simulink model "TST_Rail_MonMeUn"  (R2016b)
settings: Solver=FixedStepDiscrete  StartTime=0.0  StopTime=simTime  FixedStep=sampleTime  RelTol=1e-3
values from neighbouring files (symbols this model uses):
  testCase = 1    [initTST_Rail_MonMeUn_001.m]    (also in initTST_Rail_MonMeUn_002.m = 2; initTST_Rail_MonMeUn_003.m = 3; initTST_Rail_MonMeUn_004.m = 4; initTST_Rail_MonMeUn_005.m = 5)
libraries: simulink x91, UnitTest_Lib x81
(part 5 of 5)

== system TST_Rail_MonMeUn/compareSignals/Requirement_003/specifyOutputs ==
  sig_Req_Bus : Inport
  sig_Result_Bus : Inport  Port=2
  AndN : Logic  Inputs=9
  BS_Req : BusSelector  OutputSignals=testSig_DFC_RailMeUn0_DSM,testSig_DFC_RailMeUn2_DSM,testSig_DFC_RailMeUn22_DSM,testSig_DFC_RailMeUn3_DSM,testSig_DFC_RailMeUn4_DSM,testSig_DFC_RailMeUn42_DSM,testSig_DFC_RailMeUn7_DSM,testSig_DFC_RailMeUn8_DSM,testSig_DFC_RailMeUn10_DSM
  BS_Result : BusSelector  OutputSignals=DFC_RailMeUn0_DSM,DFC_RailMeUn2_DSM,DFC_RailMeUn22_DSM,DFC_RailMeUn3_DSM,DFC_RailMeUn4_DSM,DFC_RailMeUn42_DSM,DFC_RailMeUn7_DSM,DFC_RailMeUn8_DSM,DFC_RailMeUn10_DSM
  Bitwise_And{1..9} (9 alike) : simulink/Logic and Bit Operations/Bitwise Operator  logicop=AND  UseBitMask=off  BitMask=bin2dec('11011001')  BitMaskRealWorld=Stored Integer
  Scope : Scope  NumInputPorts=9
  Scope{1..9} (9 alike) : Scope  NumInputPorts=2
  cmp_{1..9} (9 alike) : UnitTest_Lib/RoughlyEqual  slope=0.1
  result_tws : ToWorkspace  VariableName=spec_result_003
  tws_1 : ToWorkspace  VariableName=spec_req_003_001
  tws_2 : ToWorkspace  VariableName=spec_req_003_002
  tws_3 : ToWorkspace  VariableName=spec_req_003_003
  tws_4 : ToWorkspace  VariableName=spec_req_003_004
  tws_5 : ToWorkspace  VariableName=spec_req_003_005
  tws_6 : ToWorkspace  VariableName=spec_req_003_006
  tws_7 : ToWorkspace  VariableName=spec_req_003_007
  tws_8 : ToWorkspace  VariableName=spec_req_003_008
  tws_9 : ToWorkspace  VariableName=spec_req_003_009
  result : Outport
  wires:
  sig_Req_Bus/1 -> BS_Req/1
  sig_Result_Bus/1 -> BS_Result/1
  AndN/1 -> result/1, result_tws/1
  BS_Req/1 -> cmp_1/1, Scope1/1  "<testSig_DFC_RailMeUn0_DSM>"
  BS_Result/1 -> cmp_1/2, Scope1/2  "<DFC_RailMeUn0_DSM>"
  cmp_1/1 -> Bitwise_And1/1
  Bitwise_And1/1 -> tws_1/1, AndN/1, Scope/1
  BS_Req/2 -> cmp_2/1, Scope2/1  "<testSig_DFC_RailMeUn2_DSM>"
  BS_Result/2 -> cmp_2/2, Scope2/2  "<DFC_RailMeUn2_DSM>"
  cmp_2/1 -> Bitwise_And2/1
  Bitwise_And2/1 -> tws_2/1, AndN/2, Scope/2
  BS_Req/3 -> cmp_3/1, Scope3/1  "<testSig_DFC_RailMeUn22_DSM>"
  BS_Result/3 -> cmp_3/2, Scope3/2  "<DFC_RailMeUn22_DSM>"
  cmp_3/1 -> Bitwise_And3/1
  Bitwise_And3/1 -> tws_3/1, AndN/3, Scope/3
  BS_Req/4 -> cmp_4/1, Scope4/1  "<testSig_DFC_RailMeUn3_DSM>"
  BS_Result/4 -> cmp_4/2, Scope4/2  "<DFC_RailMeUn3_DSM>"
  cmp_4/1 -> Bitwise_And4/1
  Bitwise_And4/1 -> tws_4/1, AndN/4, Scope/4
  BS_Req/5 -> cmp_5/1, Scope5/1  "<testSig_DFC_RailMeUn4_DSM>"
  BS_Result/5 -> cmp_5/2, Scope5/2  "<DFC_RailMeUn4_DSM>"
  cmp_5/1 -> Bitwise_And5/1
  Bitwise_And5/1 -> tws_5/1, AndN/5, Scope/5
  BS_Req/6 -> cmp_6/1, Scope6/1  "<testSig_DFC_RailMeUn42_DSM>"
  BS_Result/6 -> cmp_6/2, Scope6/2  "<DFC_RailMeUn42_DSM>"
  cmp_6/1 -> Bitwise_And6/1
  Bitwise_And6/1 -> tws_6/1, AndN/6, Scope/6
  BS_Req/7 -> cmp_7/1, Scope7/1  "<testSig_DFC_RailMeUn7_DSM>"
  BS_Result/7 -> cmp_7/2, Scope7/2  "<DFC_RailMeUn7_DSM>"
  cmp_7/1 -> Bitwise_And7/1
  Bitwise_And7/1 -> tws_7/1, AndN/7, Scope/7
  BS_Req/8 -> cmp_8/1, Scope8/1  "<testSig_DFC_RailMeUn8_DSM>"
  BS_Result/8 -> cmp_8/2, Scope8/2  "<DFC_RailMeUn8_DSM>"
  cmp_8/1 -> Bitwise_And8/1
  Bitwise_And8/1 -> tws_8/1, AndN/8, Scope/8
  BS_Req/9 -> cmp_9/1, Scope9/1  "<testSig_DFC_RailMeUn10_DSM>"
  BS_Result/9 -> cmp_9/2, Scope9/2  "<DFC_RailMeUn10_DSM>"
  cmp_9/1 -> Bitwise_And9/1
  Bitwise_And9/1 -> tws_9/1, AndN/9, Scope/9

== system TST_Rail_MonMeUn/compareSignals/Requirement_004/specifyOutputs ==
  sig_Req_Bus : Inport
  sig_Result_Bus : Inport  Port=2
  AndN : Logic  Inputs=9
  BS_Req : BusSelector  OutputSignals=testSig_DFC_RailMeUn0_DSM,testSig_DFC_RailMeUn2_DSM,testSig_DFC_RailMeUn22_DSM,testSig_DFC_RailMeUn3_DSM,testSig_DFC_RailMeUn4_DSM,testSig_DFC_RailMeUn42_DSM,testSig_DFC_RailMeUn7_DSM,testSig_DFC_RailMeUn8_DSM,testSig_DFC_RailMeUn10_DSM
  BS_Result : BusSelector  OutputSignals=DFC_RailMeUn0_DSM,DFC_RailMeUn2_DSM,DFC_RailMeUn22_DSM,DFC_RailMeUn3_DSM,DFC_RailMeUn4_DSM,DFC_RailMeUn42_DSM,DFC_RailMeUn7_DSM,DFC_RailMeUn8_DSM,DFC_RailMeUn10_DSM
  Bitwise_And{1..9} (9 alike) : simulink/Logic and Bit Operations/Bitwise Operator  logicop=AND  UseBitMask=off  BitMask=bin2dec('11011001')  BitMaskRealWorld=Stored Integer
  Scope : Scope  NumInputPorts=9
  Scope{1..9} (9 alike) : Scope  NumInputPorts=2
  cmp_{1..9} (9 alike) : UnitTest_Lib/RoughlyEqual  slope=0.1
  result_tws : ToWorkspace  VariableName=spec_result_004
  tws_1 : ToWorkspace  VariableName=spec_req_004_001
  tws_2 : ToWorkspace  VariableName=spec_req_004_002
  tws_3 : ToWorkspace  VariableName=spec_req_004_003
  tws_4 : ToWorkspace  VariableName=spec_req_004_004
  tws_5 : ToWorkspace  VariableName=spec_req_004_005
  tws_6 : ToWorkspace  VariableName=spec_req_004_006
  tws_7 : ToWorkspace  VariableName=spec_req_004_007
  tws_8 : ToWorkspace  VariableName=spec_req_004_008
  tws_9 : ToWorkspace  VariableName=spec_req_004_009
  result : Outport
  wires:
  sig_Req_Bus/1 -> BS_Req/1
  sig_Result_Bus/1 -> BS_Result/1
  AndN/1 -> result/1, result_tws/1
  BS_Req/1 -> cmp_1/1, Scope1/1  "<testSig_DFC_RailMeUn0_DSM>"
  BS_Result/1 -> cmp_1/2, Scope1/2  "<DFC_RailMeUn0_DSM>"
  cmp_1/1 -> Bitwise_And1/1
  Bitwise_And1/1 -> tws_1/1, AndN/1, Scope/1
  BS_Req/2 -> cmp_2/1, Scope2/1  "<testSig_DFC_RailMeUn2_DSM>"
  BS_Result/2 -> cmp_2/2, Scope2/2  "<DFC_RailMeUn2_DSM>"
  cmp_2/1 -> Bitwise_And2/1
  Bitwise_And2/1 -> tws_2/1, AndN/2, Scope/2
  BS_Req/3 -> cmp_3/1, Scope3/1  "<testSig_DFC_RailMeUn22_DSM>"
  BS_Result/3 -> cmp_3/2, Scope3/2  "<DFC_RailMeUn22_DSM>"
  cmp_3/1 -> Bitwise_And3/1
  Bitwise_And3/1 -> tws_3/1, AndN/3, Scope/3
  BS_Req/4 -> cmp_4/1, Scope4/1  "<testSig_DFC_RailMeUn3_DSM>"
  BS_Result/4 -> cmp_4/2, Scope4/2  "<DFC_RailMeUn3_DSM>"
  cmp_4/1 -> Bitwise_And4/1
  Bitwise_And4/1 -> tws_4/1, AndN/4, Scope/4
  BS_Req/5 -> cmp_5/1, Scope5/1  "<testSig_DFC_RailMeUn4_DSM>"
  BS_Result/5 -> cmp_5/2, Scope5/2  "<DFC_RailMeUn4_DSM>"
  cmp_5/1 -> Bitwise_And5/1
  Bitwise_And5/1 -> tws_5/1, AndN/5, Scope/5
  BS_Req/6 -> cmp_6/1, Scope6/1  "<testSig_DFC_RailMeUn42_DSM>"
  BS_Result/6 -> cmp_6/2, Scope6/2  "<DFC_RailMeUn42_DSM>"
  cmp_6/1 -> Bitwise_And6/1
  Bitwise_And6/1 -> tws_6/1, AndN/6, Scope/6
  BS_Req/7 -> cmp_7/1, Scope7/1  "<testSig_DFC_RailMeUn7_DSM>"
  BS_Result/7 -> cmp_7/2, Scope7/2  "<DFC_RailMeUn7_DSM>"
  cmp_7/1 -> Bitwise_And7/1
  Bitwise_And7/1 -> tws_7/1, AndN/7, Scope/7
  BS_Req/8 -> cmp_8/1, Scope8/1  "<testSig_DFC_RailMeUn8_DSM>"
  BS_Result/8 -> cmp_8/2, Scope8/2  "<DFC_RailMeUn8_DSM>"
  cmp_8/1 -> Bitwise_And8/1
  Bitwise_And8/1 -> tws_8/1, AndN/8, Scope/8
  BS_Req/9 -> cmp_9/1, Scope9/1  "<testSig_DFC_RailMeUn10_DSM>"
  BS_Result/9 -> cmp_9/2, Scope9/2  "<DFC_RailMeUn10_DSM>"
  cmp_9/1 -> Bitwise_And9/1
  Bitwise_And9/1 -> tws_9/1, AndN/9, Scope/9

== system TST_Rail_MonMeUn/compareSignals/Requirement_005/specifyOutputs ==
  sig_Req_Bus : Inport
  sig_Result_Bus : Inport  Port=2
  AndN : Logic  Inputs=9
  BS_Req : BusSelector  OutputSignals=testSig_DFC_RailMeUn0_DSM,testSig_DFC_RailMeUn2_DSM,testSig_DFC_RailMeUn22_DSM,testSig_DFC_RailMeUn3_DSM,testSig_DFC_RailMeUn4_DSM,testSig_DFC_RailMeUn42_DSM,testSig_DFC_RailMeUn7_DSM,testSig_DFC_RailMeUn8_DSM,testSig_DFC_RailMeUn10_DSM
  BS_Result : BusSelector  OutputSignals=DFC_RailMeUn0_DSM,DFC_RailMeUn2_DSM,DFC_RailMeUn22_DSM,DFC_RailMeUn3_DSM,DFC_RailMeUn4_DSM,DFC_RailMeUn42_DSM,DFC_RailMeUn7_DSM,DFC_RailMeUn8_DSM,DFC_RailMeUn10_DSM
  Bitwise_And{1..9} (9 alike) : simulink/Logic and Bit Operations/Bitwise Operator  logicop=AND  UseBitMask=off  BitMask=bin2dec('11011001')  BitMaskRealWorld=Stored Integer
  Scope : Scope  NumInputPorts=9
  Scope{1..9} (9 alike) : Scope  NumInputPorts=2
  cmp_{1..9} (9 alike) : UnitTest_Lib/RoughlyEqual  slope=0.1
  result_tws : ToWorkspace  VariableName=spec_result_005
  tws_1 : ToWorkspace  VariableName=spec_req_005_001
  tws_2 : ToWorkspace  VariableName=spec_req_005_002
  tws_3 : ToWorkspace  VariableName=spec_req_005_003
  tws_4 : ToWorkspace  VariableName=spec_req_005_004
  tws_5 : ToWorkspace  VariableName=spec_req_005_005
  tws_6 : ToWorkspace  VariableName=spec_req_005_006
  tws_7 : ToWorkspace  VariableName=spec_req_005_007
  tws_8 : ToWorkspace  VariableName=spec_req_005_008
  tws_9 : ToWorkspace  VariableName=spec_req_005_009
  result : Outport
  wires:
  sig_Req_Bus/1 -> BS_Req/1
  sig_Result_Bus/1 -> BS_Result/1
  AndN/1 -> result/1, result_tws/1
  BS_Req/1 -> cmp_1/1, Scope1/1  "<testSig_DFC_RailMeUn0_DSM>"
  BS_Result/1 -> cmp_1/2, Scope1/2  "<DFC_RailMeUn0_DSM>"
  cmp_1/1 -> Bitwise_And1/1
  Bitwise_And1/1 -> tws_1/1, AndN/1, Scope/1
  BS_Req/2 -> cmp_2/1, Scope2/1  "<testSig_DFC_RailMeUn2_DSM>"
  BS_Result/2 -> cmp_2/2, Scope2/2  "<DFC_RailMeUn2_DSM>"
  cmp_2/1 -> Bitwise_And2/1
  Bitwise_And2/1 -> tws_2/1, AndN/2, Scope/2
  BS_Req/3 -> cmp_3/1, Scope3/1  "<testSig_DFC_RailMeUn22_DSM>"
  BS_Result/3 -> cmp_3/2, Scope3/2  "<DFC_RailMeUn22_DSM>"
  cmp_3/1 -> Bitwise_And3/1
  Bitwise_And3/1 -> tws_3/1, AndN/3, Scope/3
  BS_Req/4 -> cmp_4/1, Scope4/1  "<testSig_DFC_RailMeUn3_DSM>"
  BS_Result/4 -> cmp_4/2, Scope4/2  "<DFC_RailMeUn3_DSM>"
  cmp_4/1 -> Bitwise_And4/1
  Bitwise_And4/1 -> tws_4/1, AndN/4, Scope/4
  BS_Req/5 -> cmp_5/1, Scope5/1  "<testSig_DFC_RailMeUn4_DSM>"
  BS_Result/5 -> cmp_5/2, Scope5/2  "<DFC_RailMeUn4_DSM>"
  cmp_5/1 -> Bitwise_And5/1
  Bitwise_And5/1 -> tws_5/1, AndN/5, Scope/5
  BS_Req/6 -> cmp_6/1, Scope6/1  "<testSig_DFC_RailMeUn42_DSM>"
  BS_Result/6 -> cmp_6/2, Scope6/2  "<DFC_RailMeUn42_DSM>"
  cmp_6/1 -> Bitwise_And6/1
  Bitwise_And6/1 -> tws_6/1, AndN/6, Scope/6
  BS_Req/7 -> cmp_7/1, Scope7/1  "<testSig_DFC_RailMeUn7_DSM>"
  BS_Result/7 -> cmp_7/2, Scope7/2  "<DFC_RailMeUn7_DSM>"
  cmp_7/1 -> Bitwise_And7/1
  Bitwise_And7/1 -> tws_7/1, AndN/7, Scope/7
  BS_Req/8 -> cmp_8/1, Scope8/1  "<testSig_DFC_RailMeUn8_DSM>"
  BS_Result/8 -> cmp_8/2, Scope8/2  "<DFC_RailMeUn8_DSM>"
  cmp_8/1 -> Bitwise_And8/1
  Bitwise_And8/1 -> tws_8/1, AndN/8, Scope/8
  BS_Req/9 -> cmp_9/1, Scope9/1  "<testSig_DFC_RailMeUn10_DSM>"
  BS_Result/9 -> cmp_9/2, Scope9/2  "<DFC_RailMeUn10_DSM>"
  cmp_9/1 -> Bitwise_And9/1
  Bitwise_And9/1 -> tws_9/1, AndN/9, Scope/9

== system TST_Rail_MonMeUn/compareSignals/Requirement_006/specifyOutputs ==
  sig_Req_Bus : Inport
  sig_Result_Bus : Inport  Port=2
  AndN : Logic  Inputs=9
  BS_Req : BusSelector  OutputSignals=testSig_DFC_RailMeUn0_DSM,testSig_DFC_RailMeUn2_DSM,testSig_DFC_RailMeUn22_DSM,testSig_DFC_RailMeUn3_DSM,testSig_DFC_RailMeUn4_DSM,testSig_DFC_RailMeUn42_DSM,testSig_DFC_RailMeUn7_DSM,testSig_DFC_RailMeUn8_DSM,testSig_DFC_RailMeUn10_DSM
  BS_Result : BusSelector  OutputSignals=DFC_RailMeUn0_DSM,DFC_RailMeUn2_DSM,DFC_RailMeUn22_DSM,DFC_RailMeUn3_DSM,DFC_RailMeUn4_DSM,DFC_RailMeUn42_DSM,DFC_RailMeUn7_DSM,DFC_RailMeUn8_DSM,DFC_RailMeUn10_DSM
  Bitwise_And{1..9} (9 alike) : simulink/Logic and Bit Operations/Bitwise Operator  logicop=AND  UseBitMask=off  BitMask=bin2dec('11011001')  BitMaskRealWorld=Stored Integer
  Scope : Scope  NumInputPorts=9
  Scope{1..9} (9 alike) : Scope  NumInputPorts=2
  cmp_{1..9} (9 alike) : UnitTest_Lib/RoughlyEqual  slope=0.1
  result_tws : ToWorkspace  VariableName=spec_result_006
  tws_1 : ToWorkspace  VariableName=spec_req_006_001
  tws_2 : ToWorkspace  VariableName=spec_req_006_002
  tws_3 : ToWorkspace  VariableName=spec_req_006_003
  tws_4 : ToWorkspace  VariableName=spec_req_006_004
  tws_5 : ToWorkspace  VariableName=spec_req_006_005
  tws_6 : ToWorkspace  VariableName=spec_req_006_006
  tws_7 : ToWorkspace  VariableName=spec_req_006_007
  tws_8 : ToWorkspace  VariableName=spec_req_006_008
  tws_9 : ToWorkspace  VariableName=spec_req_006_009
  result : Outport
  wires:
  sig_Req_Bus/1 -> BS_Req/1
  sig_Result_Bus/1 -> BS_Result/1
  AndN/1 -> result/1, result_tws/1
  BS_Req/1 -> cmp_1/1, Scope1/1  "<testSig_DFC_RailMeUn0_DSM>"
  BS_Result/1 -> cmp_1/2, Scope1/2  "<DFC_RailMeUn0_DSM>"
  cmp_1/1 -> Bitwise_And1/1
  Bitwise_And1/1 -> tws_1/1, AndN/1, Scope/1
  BS_Req/2 -> cmp_2/1, Scope2/1  "<testSig_DFC_RailMeUn2_DSM>"
  BS_Result/2 -> cmp_2/2, Scope2/2  "<DFC_RailMeUn2_DSM>"
  cmp_2/1 -> Bitwise_And2/1
  Bitwise_And2/1 -> tws_2/1, AndN/2, Scope/2
  BS_Req/3 -> cmp_3/1, Scope3/1  "<testSig_DFC_RailMeUn22_DSM>"
  BS_Result/3 -> cmp_3/2, Scope3/2  "<DFC_RailMeUn22_DSM>"
  cmp_3/1 -> Bitwise_And3/1
  Bitwise_And3/1 -> tws_3/1, AndN/3, Scope/3
  BS_Req/4 -> cmp_4/1, Scope4/1  "<testSig_DFC_RailMeUn3_DSM>"
  BS_Result/4 -> cmp_4/2, Scope4/2  "<DFC_RailMeUn3_DSM>"
  cmp_4/1 -> Bitwise_And4/1
  Bitwise_And4/1 -> tws_4/1, AndN/4, Scope/4
  BS_Req/5 -> cmp_5/1, Scope5/1  "<testSig_DFC_RailMeUn4_DSM>"
  BS_Result/5 -> cmp_5/2, Scope5/2  "<DFC_RailMeUn4_DSM>"
  cmp_5/1 -> Bitwise_And5/1
  Bitwise_And5/1 -> tws_5/1, AndN/5, Scope/5
  BS_Req/6 -> cmp_6/1, Scope6/1  "<testSig_DFC_RailMeUn42_DSM>"
  BS_Result/6 -> cmp_6/2, Scope6/2  "<DFC_RailMeUn42_DSM>"
  cmp_6/1 -> Bitwise_And6/1
  Bitwise_And6/1 -> tws_6/1, AndN/6, Scope/6
  BS_Req/7 -> cmp_7/1, Scope7/1  "<testSig_DFC_RailMeUn7_DSM>"
  BS_Result/7 -> cmp_7/2, Scope7/2  "<DFC_RailMeUn7_DSM>"
  cmp_7/1 -> Bitwise_And7/1
  Bitwise_And7/1 -> tws_7/1, AndN/7, Scope/7
  BS_Req/8 -> cmp_8/1, Scope8/1  "<testSig_DFC_RailMeUn8_DSM>"
  BS_Result/8 -> cmp_8/2, Scope8/2  "<DFC_RailMeUn8_DSM>"
  cmp_8/1 -> Bitwise_And8/1
  Bitwise_And8/1 -> tws_8/1, AndN/8, Scope/8
  BS_Req/9 -> cmp_9/1, Scope9/1  "<testSig_DFC_RailMeUn10_DSM>"
  BS_Result/9 -> cmp_9/2, Scope9/2  "<DFC_RailMeUn10_DSM>"
  cmp_9/1 -> Bitwise_And9/1
  Bitwise_And9/1 -> tws_9/1, AndN/9, Scope/9

== system TST_Rail_MonMeUn/compareSignals/Requirement_007/specifyOutputs ==
  sig_Req_Bus : Inport
  sig_Result_Bus : Inport  Port=2
  AndN : Logic  Inputs=9
  BS_Req : BusSelector  OutputSignals=testSig_DFC_RailMeUn0_DSM,testSig_DFC_RailMeUn2_DSM,testSig_DFC_RailMeUn22_DSM,testSig_DFC_RailMeUn3_DSM,testSig_DFC_RailMeUn4_DSM,testSig_DFC_RailMeUn42_DSM,testSig_DFC_RailMeUn7_DSM,testSig_DFC_RailMeUn8_DSM,testSig_DFC_RailMeUn10_DSM
  BS_Result : BusSelector  OutputSignals=DFC_RailMeUn0_DSM,DFC_RailMeUn2_DSM,DFC_RailMeUn22_DSM,DFC_RailMeUn3_DSM,DFC_RailMeUn4_DSM,DFC_RailMeUn42_DSM,DFC_RailMeUn7_DSM,DFC_RailMeUn8_DSM,DFC_RailMeUn10_DSM
  Bitwise_And{1..9} (9 alike) : simulink/Logic and Bit Operations/Bitwise Operator  logicop=AND  UseBitMask=off  BitMask=bin2dec('11011001')  BitMaskRealWorld=Stored Integer
  Scope : Scope  NumInputPorts=9
  Scope{1..9} (9 alike) : Scope  NumInputPorts=2
  cmp_{1..9} (9 alike) : UnitTest_Lib/RoughlyEqual  slope=0.1
  result_tws : ToWorkspace  VariableName=spec_result_007
  tws_1 : ToWorkspace  VariableName=spec_req_007_001
  tws_2 : ToWorkspace  VariableName=spec_req_007_002
  tws_3 : ToWorkspace  VariableName=spec_req_007_003
  tws_4 : ToWorkspace  VariableName=spec_req_007_004
  tws_5 : ToWorkspace  VariableName=spec_req_007_005
  tws_6 : ToWorkspace  VariableName=spec_req_007_006
  tws_7 : ToWorkspace  VariableName=spec_req_007_007
  tws_8 : ToWorkspace  VariableName=spec_req_007_008
  tws_9 : ToWorkspace  VariableName=spec_req_007_009
  result : Outport
  wires:
  sig_Req_Bus/1 -> BS_Req/1
  sig_Result_Bus/1 -> BS_Result/1
  AndN/1 -> result/1, result_tws/1
  BS_Req/1 -> cmp_1/1, Scope1/1  "<testSig_DFC_RailMeUn0_DSM>"
  BS_Result/1 -> cmp_1/2, Scope1/2  "<DFC_RailMeUn0_DSM>"
  cmp_1/1 -> Bitwise_And1/1
  Bitwise_And1/1 -> tws_1/1, AndN/1, Scope/1
  BS_Req/2 -> cmp_2/1, Scope2/1  "<testSig_DFC_RailMeUn2_DSM>"
  BS_Result/2 -> cmp_2/2, Scope2/2  "<DFC_RailMeUn2_DSM>"
  cmp_2/1 -> Bitwise_And2/1
  Bitwise_And2/1 -> tws_2/1, AndN/2, Scope/2
  BS_Req/3 -> cmp_3/1, Scope3/1  "<testSig_DFC_RailMeUn22_DSM>"
  BS_Result/3 -> cmp_3/2, Scope3/2  "<DFC_RailMeUn22_DSM>"
  cmp_3/1 -> Bitwise_And3/1
  Bitwise_And3/1 -> tws_3/1, AndN/3, Scope/3
  BS_Req/4 -> cmp_4/1, Scope4/1  "<testSig_DFC_RailMeUn3_DSM>"
  BS_Result/4 -> cmp_4/2, Scope4/2  "<DFC_RailMeUn3_DSM>"
  cmp_4/1 -> Bitwise_And4/1
  Bitwise_And4/1 -> tws_4/1, AndN/4, Scope/4
  BS_Req/5 -> cmp_5/1, Scope5/1  "<testSig_DFC_RailMeUn4_DSM>"
  BS_Result/5 -> cmp_5/2, Scope5/2  "<DFC_RailMeUn4_DSM>"
  cmp_5/1 -> Bitwise_And5/1
  Bitwise_And5/1 -> tws_5/1, AndN/5, Scope/5
  BS_Req/6 -> cmp_6/1, Scope6/1  "<testSig_DFC_RailMeUn42_DSM>"
  BS_Result/6 -> cmp_6/2, Scope6/2  "<DFC_RailMeUn42_DSM>"
  cmp_6/1 -> Bitwise_And6/1
  Bitwise_And6/1 -> tws_6/1, AndN/6, Scope/6
  BS_Req/7 -> cmp_7/1, Scope7/1  "<testSig_DFC_RailMeUn7_DSM>"
  BS_Result/7 -> cmp_7/2, Scope7/2  "<DFC_RailMeUn7_DSM>"
  cmp_7/1 -> Bitwise_And7/1
  Bitwise_And7/1 -> tws_7/1, AndN/7, Scope/7
  BS_Req/8 -> cmp_8/1, Scope8/1  "<testSig_DFC_RailMeUn8_DSM>"
  BS_Result/8 -> cmp_8/2, Scope8/2  "<DFC_RailMeUn8_DSM>"
  cmp_8/1 -> Bitwise_And8/1
  Bitwise_And8/1 -> tws_8/1, AndN/8, Scope/8
  BS_Req/9 -> cmp_9/1, Scope9/1  "<testSig_DFC_RailMeUn10_DSM>"
  BS_Result/9 -> cmp_9/2, Scope9/2  "<DFC_RailMeUn10_DSM>"
  cmp_9/1 -> Bitwise_And9/1
  Bitwise_And9/1 -> tws_9/1, AndN/9, Scope/9

== system TST_Rail_MonMeUn/compareSignals/Requirement_008/specifyOutputs ==
  sig_Req_Bus : Inport
  sig_Result_Bus : Inport  Port=2
  AndN : Logic  Inputs=9
  BS_Req : BusSelector  OutputSignals=testSig_DFC_RailMeUn0_DSM,testSig_DFC_RailMeUn2_DSM,testSig_DFC_RailMeUn22_DSM,testSig_DFC_RailMeUn3_DSM,testSig_DFC_RailMeUn4_DSM,testSig_DFC_RailMeUn42_DSM,testSig_DFC_RailMeUn7_DSM,testSig_DFC_RailMeUn8_DSM,testSig_DFC_RailMeUn10_DSM
  BS_Result : BusSelector  OutputSignals=DFC_RailMeUn0_DSM,DFC_RailMeUn2_DSM,DFC_RailMeUn22_DSM,DFC_RailMeUn3_DSM,DFC_RailMeUn4_DSM,DFC_RailMeUn42_DSM,DFC_RailMeUn7_DSM,DFC_RailMeUn8_DSM,DFC_RailMeUn10_DSM
  Bitwise_And{1..9} (9 alike) : simulink/Logic and Bit Operations/Bitwise Operator  logicop=AND  UseBitMask=off  BitMask=bin2dec('11011001')  BitMaskRealWorld=Stored Integer
  Scope : Scope  NumInputPorts=9
  Scope{1..9} (9 alike) : Scope  NumInputPorts=2
  cmp_{1..9} (9 alike) : UnitTest_Lib/RoughlyEqual  slope=0.1
  result_tws : ToWorkspace  VariableName=spec_result_008
  tws_1 : ToWorkspace  VariableName=spec_req_008_001
  tws_2 : ToWorkspace  VariableName=spec_req_008_002
  tws_3 : ToWorkspace  VariableName=spec_req_008_003
  tws_4 : ToWorkspace  VariableName=spec_req_008_004
  tws_5 : ToWorkspace  VariableName=spec_req_008_005
  tws_6 : ToWorkspace  VariableName=spec_req_008_006
  tws_7 : ToWorkspace  VariableName=spec_req_008_007
  tws_8 : ToWorkspace  VariableName=spec_req_008_008
  tws_9 : ToWorkspace  VariableName=spec_req_008_009
  result : Outport
  wires:
  sig_Req_Bus/1 -> BS_Req/1
  sig_Result_Bus/1 -> BS_Result/1
  AndN/1 -> result/1, result_tws/1
  BS_Req/1 -> cmp_1/1, Scope1/1  "<testSig_DFC_RailMeUn0_DSM>"
  BS_Result/1 -> cmp_1/2, Scope1/2  "<DFC_RailMeUn0_DSM>"
  cmp_1/1 -> Bitwise_And1/1
  Bitwise_And1/1 -> tws_1/1, AndN/1, Scope/1
  BS_Req/2 -> cmp_2/1, Scope2/1  "<testSig_DFC_RailMeUn2_DSM>"
  BS_Result/2 -> cmp_2/2, Scope2/2  "<DFC_RailMeUn2_DSM>"
  cmp_2/1 -> Bitwise_And2/1
  Bitwise_And2/1 -> tws_2/1, AndN/2, Scope/2
  BS_Req/3 -> cmp_3/1, Scope3/1  "<testSig_DFC_RailMeUn22_DSM>"
  BS_Result/3 -> cmp_3/2, Scope3/2  "<DFC_RailMeUn22_DSM>"
  cmp_3/1 -> Bitwise_And3/1
  Bitwise_And3/1 -> tws_3/1, AndN/3, Scope/3
  BS_Req/4 -> cmp_4/1, Scope4/1  "<testSig_DFC_RailMeUn3_DSM>"
  BS_Result/4 -> cmp_4/2, Scope4/2  "<DFC_RailMeUn3_DSM>"
  cmp_4/1 -> Bitwise_And4/1
  Bitwise_And4/1 -> tws_4/1, AndN/4, Scope/4
  BS_Req/5 -> cmp_5/1, Scope5/1  "<testSig_DFC_RailMeUn4_DSM>"
  BS_Result/5 -> cmp_5/2, Scope5/2  "<DFC_RailMeUn4_DSM>"
  cmp_5/1 -> Bitwise_And5/1
  Bitwise_And5/1 -> tws_5/1, AndN/5, Scope/5
  BS_Req/6 -> cmp_6/1, Scope6/1  "<testSig_DFC_RailMeUn42_DSM>"
  BS_Result/6 -> cmp_6/2, Scope6/2  "<DFC_RailMeUn42_DSM>"
  cmp_6/1 -> Bitwise_And6/1
  Bitwise_And6/1 -> tws_6/1, AndN/6, Scope/6
  BS_Req/7 -> cmp_7/1, Scope7/1  "<testSig_DFC_RailMeUn7_DSM>"
  BS_Result/7 -> cmp_7/2, Scope7/2  "<DFC_RailMeUn7_DSM>"
  cmp_7/1 -> Bitwise_And7/1
  Bitwise_And7/1 -> tws_7/1, AndN/7, Scope/7
  BS_Req/8 -> cmp_8/1, Scope8/1  "<testSig_DFC_RailMeUn8_DSM>"
  BS_Result/8 -> cmp_8/2, Scope8/2  "<DFC_RailMeUn8_DSM>"
  cmp_8/1 -> Bitwise_And8/1
  Bitwise_And8/1 -> tws_8/1, AndN/8, Scope/8
  BS_Req/9 -> cmp_9/1, Scope9/1  "<testSig_DFC_RailMeUn10_DSM>"
  BS_Result/9 -> cmp_9/2, Scope9/2  "<DFC_RailMeUn10_DSM>"
  cmp_9/1 -> Bitwise_And9/1
  Bitwise_And9/1 -> tws_9/1, AndN/9, Scope/9

== system TST_Rail_MonMeUn/compareSignals/Requirement_009/specifyOutputs ==
  sig_Req_Bus : Inport
  sig_Result_Bus : Inport  Port=2
  AndN : Logic  Inputs=9
  BS_Req : BusSelector  OutputSignals=testSig_DFC_RailMeUn0_DSM,testSig_DFC_RailMeUn2_DSM,testSig_DFC_RailMeUn22_DSM,testSig_DFC_RailMeUn3_DSM,testSig_DFC_RailMeUn4_DSM,testSig_DFC_RailMeUn42_DSM,testSig_DFC_RailMeUn7_DSM,testSig_DFC_RailMeUn8_DSM,testSig_DFC_RailMeUn10_DSM
  BS_Result : BusSelector  OutputSignals=DFC_RailMeUn0_DSM,DFC_RailMeUn2_DSM,DFC_RailMeUn22_DSM,DFC_RailMeUn3_DSM,DFC_RailMeUn4_DSM,DFC_RailMeUn42_DSM,DFC_RailMeUn7_DSM,DFC_RailMeUn8_DSM,DFC_RailMeUn10_DSM
  Bitwise_And{1..9} (9 alike) : simulink/Logic and Bit Operations/Bitwise Operator  logicop=AND  UseBitMask=off  BitMask=bin2dec('11011001')  BitMaskRealWorld=Stored Integer
  Scope : Scope  NumInputPorts=9
  Scope{1..9} (9 alike) : Scope  NumInputPorts=2
  cmp_{1..9} (9 alike) : UnitTest_Lib/RoughlyEqual  slope=0.1
  result_tws : ToWorkspace  VariableName=spec_result_009
  tws_1 : ToWorkspace  VariableName=spec_req_009_001
  tws_2 : ToWorkspace  VariableName=spec_req_009_002
  tws_3 : ToWorkspace  VariableName=spec_req_009_003
  tws_4 : ToWorkspace  VariableName=spec_req_009_004
  tws_5 : ToWorkspace  VariableName=spec_req_009_005
  tws_6 : ToWorkspace  VariableName=spec_req_009_006
  tws_7 : ToWorkspace  VariableName=spec_req_009_007
  tws_8 : ToWorkspace  VariableName=spec_req_009_008
  tws_9 : ToWorkspace  VariableName=spec_req_009_009
  result : Outport
  wires:
  sig_Req_Bus/1 -> BS_Req/1
  sig_Result_Bus/1 -> BS_Result/1
  AndN/1 -> result/1, result_tws/1
  BS_Req/1 -> cmp_1/1, Scope1/1  "<testSig_DFC_RailMeUn0_DSM>"
  BS_Result/1 -> cmp_1/2, Scope1/2  "<DFC_RailMeUn0_DSM>"
  cmp_1/1 -> Bitwise_And1/1
  Bitwise_And1/1 -> tws_1/1, AndN/1, Scope/1
  BS_Req/2 -> cmp_2/1, Scope2/1  "<testSig_DFC_RailMeUn2_DSM>"
  BS_Result/2 -> cmp_2/2, Scope2/2  "<DFC_RailMeUn2_DSM>"
  cmp_2/1 -> Bitwise_And2/1
  Bitwise_And2/1 -> tws_2/1, AndN/2, Scope/2
  BS_Req/3 -> cmp_3/1, Scope3/1  "<testSig_DFC_RailMeUn22_DSM>"
  BS_Result/3 -> cmp_3/2, Scope3/2  "<DFC_RailMeUn22_DSM>"
  cmp_3/1 -> Bitwise_And3/1
  Bitwise_And3/1 -> tws_3/1, AndN/3, Scope/3
  BS_Req/4 -> cmp_4/1, Scope4/1  "<testSig_DFC_RailMeUn3_DSM>"
  BS_Result/4 -> cmp_4/2, Scope4/2  "<DFC_RailMeUn3_DSM>"
  cmp_4/1 -> Bitwise_And4/1
  Bitwise_And4/1 -> tws_4/1, AndN/4, Scope/4
  BS_Req/5 -> cmp_5/1, Scope5/1  "<testSig_DFC_RailMeUn4_DSM>"
  BS_Result/5 -> cmp_5/2, Scope5/2  "<DFC_RailMeUn4_DSM>"
  cmp_5/1 -> Bitwise_And5/1
  Bitwise_And5/1 -> tws_5/1, AndN/5, Scope/5
  BS_Req/6 -> cmp_6/1, Scope6/1  "<testSig_DFC_RailMeUn42_DSM>"
  BS_Result/6 -> cmp_6/2, Scope6/2  "<DFC_RailMeUn42_DSM>"
  cmp_6/1 -> Bitwise_And6/1
  Bitwise_And6/1 -> tws_6/1, AndN/6, Scope/6
  BS_Req/7 -> cmp_7/1, Scope7/1  "<testSig_DFC_RailMeUn7_DSM>"
  BS_Result/7 -> cmp_7/2, Scope7/2  "<DFC_RailMeUn7_DSM>"
  cmp_7/1 -> Bitwise_And7/1
  Bitwise_And7/1 -> tws_7/1, AndN/7, Scope/7
  BS_Req/8 -> cmp_8/1, Scope8/1  "<testSig_DFC_RailMeUn8_DSM>"
  BS_Result/8 -> cmp_8/2, Scope8/2  "<DFC_RailMeUn8_DSM>"
  cmp_8/1 -> Bitwise_And8/1
  Bitwise_And8/1 -> tws_8/1, AndN/8, Scope/8
  BS_Req/9 -> cmp_9/1, Scope9/1  "<testSig_DFC_RailMeUn10_DSM>"
  BS_Result/9 -> cmp_9/2, Scope9/2  "<DFC_RailMeUn10_DSM>"
  cmp_9/1 -> Bitwise_And9/1
  Bitwise_And9/1 -> tws_9/1, AndN/9, Scope/9
